simulink model "HDLModulatorFull"  (R2024a)
settings: Solver=FixedStepDiscrete  StartTime=0.0  StopTime=stopTime  RelTol=1e-3
values from neighbouring files (symbols this model uses):
  dataSymbols = [ ... (first row only)    [testModulatorFull.m]
undefined symbols (not defined in the file or in its folder): CONST
libraries: hdlsllib x10, dspsrcs4 x9, simulink x2, HDL_ieee_8021513 x2, whdlutilities x1
settings Model: DataTypeOverride=Off  SimulationMode=accelerator  Creator=cotti  LastModifiedBy=cotti
settings OptimizationCC: BlockReduction=off  ConditionallyExecuteInputs=off  DefaultParameterBehavior=Inlined  InheritOutputTypeSmallerThanSingle=on
settings DebuggingCC: AlgebraicLoopMsg=error  ArtificialAlgebraicLoopMsg=error  SingleTaskRateTransMsg=error  UnconnectedInputMsg=warning  UnconnectedOutputMsg=warning  UnconnectedLineMsg=warning
settings HardwareCC: ProdBitPerPointer=32  ProdBitPerSizeT=32  ProdBitPerPtrDiffT=32  ProdLargestAtomicFloat=None  ProdIntDivRoundTo=Undefined  ProdEndianess=Unspecified  ProdWordSize=32  ProdHWDeviceType=ASIC/FPGA->ASIC/FPGA  TargetBitPerLong=64  TargetBitPerPointer=64  TargetBitPerSizeT=64  TargetBitPerPtrDiffT=64  TargetLongLongMode=on  TargetIntDivRoundTo=Zero  TargetEndianess=LittleEndian  TargetWordSize=64  TargetHWDeviceType=Custom Processor->MATLAB Host Computer  ProdEqTarget=off

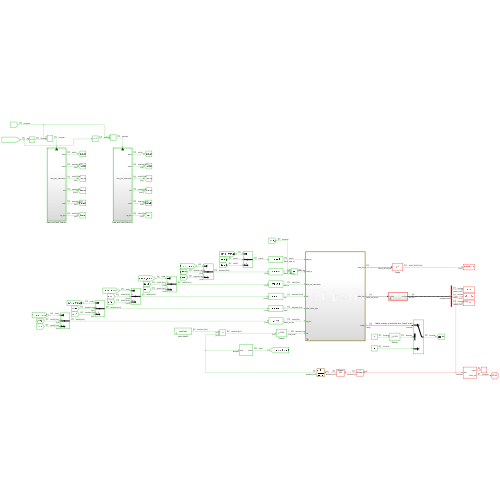
[thumbnail: Simulink's stored preview of the top-level diagram]
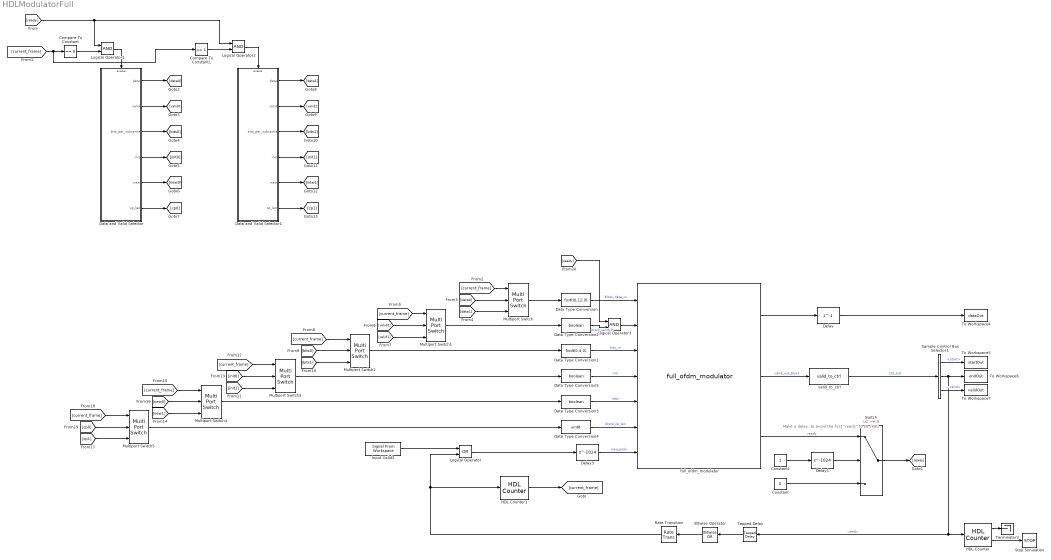
== system HDLModulatorFull ==
  note: Make a delay, to avoid the first "ready" to be read
  Bitwise Operator : simulink/Logic and Bit Operations/Bitwise Operator  logicop=OR  UseBitMask=off  BitMask=bin2dec('11011001')  BitMaskRealWorld=Stored Integer
      settings: LibrarySourceBlock=|
      | hdlsllib/Logic and Bit
      | Operations/Bitwise
      | Operator
  Compare To Constant : hdlsllib/Logic and Bit Operations/Compare To Constant  relop===  const=0  OutDataTypeStr=boolean
  Compare To Constant1 : hdlsllib/Logic and Bit Operations/Compare To Constant  relop===  const=1  OutDataTypeStr=boolean
  Constant : Constant  Value=0  OutDataTypeStr=boolean  SampleTime=1/CONST.fPHY
  Constant1 : Constant  OutDataTypeStr=boolean  SampleTime=1/CONST.fPHY
  Data Type Conversion : DataTypeConversion  OutDataTypeStr=fixdt(0,12,0)  SaturateOnIntegerOverflow=off  RndMeth=Floor  LockScale=on
  Data Type Conversion1 : DataTypeConversion  OutDataTypeStr=fixdt(0,4,0)  SaturateOnIntegerOverflow=off  RndMeth=Floor  LockScale=on
  Data Type Conversion2 : DataTypeConversion  OutDataTypeStr=boolean  SaturateOnIntegerOverflow=off  RndMeth=Floor  LockScale=on
  Data Type Conversion3 : DataTypeConversion  OutDataTypeStr=boolean  SaturateOnIntegerOverflow=off  RndMeth=Floor  LockScale=on
  Data Type Conversion4 : DataTypeConversion  OutDataTypeStr=uint8  SaturateOnIntegerOverflow=off  RndMeth=Floor  LockScale=on
  Data Type Conversion5 : DataTypeConversion  OutDataTypeStr=boolean  SaturateOnIntegerOverflow=off  RndMeth=Floor  LockScale=on
  Data and Valid Selector : Subsystem  TreatAsAtomicUnit=on
  Data and Valid Selector1 : Subsystem  TreatAsAtomicUnit=on
  Delay : Delay  DelayLength=1  InitialCondition=0  UseCircularBuffer=on
  Delay1 : Delay  DelayLength=1024  InitialCondition=0  UseCircularBuffer=on
  Delay3 : Delay  DelayLength=1024  InitialCondition=0  UseCircularBuffer=on
  HDL Counter : hdlsllib/Sources/HDL Counter  CountType=Count limited  CountInit=0  CountStep=1  CountMax=numberOfRepetitions  CountFromType=Initial value  CountFrom=0  CountResetPort=off  CountLoadPort=off  CountEnbPort=on  CountDirPort=off  CountHitOutputPort=on  CountDataType=Unsigned  CountWordLen=8  CountFracLen=0  CountSampTime=1
  HDL Counter1 : hdlsllib/Sources/HDL Counter  CountType=Free running  CountInit=0  CountStep=1  CountMax=25  CountFromType=Initial value  CountFrom=0  CountResetPort=off  CountLoadPort=off  CountEnbPort=on  CountDirPort=off  CountHitOutputPort=off  CountDataType=Unsigned  CountWordLen=8  CountFracLen=0  CountSampTime=1
  Input Valid3 : dspsrcs4/Signal From Workspace  X=newPsdu  Ts=1/CONST.fPHY  nsamps=1  OutputAfterFinalValue=Setting to zero  ignoreOrWarnInputAndFrameLengths=off  OutputFrames=off
  Logical Operator : Logic  Operator=OR  AllPortsSameDT=off  OutDataTypeStr=boolean
  Logical Operator1 : Logic  AllPortsSameDT=off  OutDataTypeStr=boolean
  Logical Operator2 : Logic  AllPortsSameDT=off  OutDataTypeStr=boolean
  Logical Operator3 : Logic  AllPortsSameDT=off  OutDataTypeStr=boolean
  Multiport Switch{,1..5} (6 alike) : MultiPortSwitch  DataPortOrder=Zero-based contiguous  Inputs=2  zeroidx=on  SaturateOnIntegerOverflow=off  InputSameDT=off
  Rate Transition : RateTransition  OutPortSampleTimeOpt=Multiple of input port sample time  OutPortSampleTimeMultiple=2
  Sample Control Bus Selector1 : whdlutilities/Sample Control Bus Selector  OutputSignals=start,end,valid
  Stop Simulation : Stop
  Switch : Switch  Criteria=u2 ~= 0  SaturateOnIntegerOverflow=off  InputSameDT=off
  Tapped Delay : simulink/Discrete/Tapped Delay  vinit=0.0  samptime=-1  NumDelays=2  DelayOrder=Oldest  includeCurrent=off
      settings: LibrarySourceBlock=hdlsllib/Discrete/Tapped Delay
  Terminator2 : Terminator
  To Workspace4 : ToWorkspace  VariableName=dataOut  SampleTime=1/CONST.fDAC
      settings: Save2DSignal=2-D array (concatenate along first dimension)
  To Workspace5 : ToWorkspace  VariableName=startOut  SampleTime=1/CONST.fDAC
      settings: Save2DSignal=2-D array (concatenate along first dimension)
  To Workspace6 : ToWorkspace  VariableName=endOut  SampleTime=1/CONST.fDAC
      settings: Save2DSignal=2-D array (concatenate along first dimension)
  To Workspace7 : ToWorkspace  VariableName=validOut  SampleTime=1/CONST.fDAC
      settings: Save2DSignal=2-D array (concatenate along first dimension)
  full_ofdm_modulator : HDL_ieee_8021513/full_ofdm_modulator  SystemSampleTime=-1  VariantActivationTime=update diagram  AllowFlexibleInterface=on  Latency=0  AutoFrameSizeCalculation=off
      settings: SourceProductName=HDL IEEE 8021513
  valid_to_ctrl : HDL_ieee_8021513/valid_to_ctrl  SystemSampleTime=-1  VariantActivationTime=update diagram  AllowFlexibleInterface=on  Latency=0  AutoFrameSizeCalculation=off
      settings: SourceProductName=HDL IEEE 8021513
  wires:
  full_ofdm_modulator/2 -> valid_to_ctrl/1  "valid_out_block"
  full_ofdm_modulator/1 -> Delay/1
  Sample Control Bus Selector1/3 -> To Workspace7/1  "<valid>"
  valid_to_ctrl/1 -> Sample Control Bus Selector1/1  "ctrl_out"
  Sample Control Bus Selector1/1 -> To Workspace5/1  "<start>"
  Sample Control Bus Selector1/2 -> Tapped Delay/1, HDL Counter/1, To Workspace6/1  "<end>"
  Data Type Conversion1/1 -> full_ofdm_modulator/3  "bits_in"
  Data Type Conversion4/1 -> full_ofdm_modulator/6  "block_cp_len"
  Data Type Conversion/1 -> full_ofdm_modulator/1  "block_data_in"
  Data Type Conversion3/1 -> full_ofdm_modulator/5  "new"
  Data Type Conversion5/1 -> full_ofdm_modulator/4  "init"
  Delay/1 -> To Workspace4/1
  HDL Counter/1 -> Terminator2/1
  HDL Counter/2 -> Stop Simulation/1
  full_ofdm_modulator/3 -> Switch/1  "ready"
  Constant/1 -> Switch/3
  Constant1/1 -> Delay1/1
  Delay1/1 -> Switch/2
  Rate Transition/1 -> Logical Operator/2, HDL Counter1/1
  Tapped Delay/1 -> Bitwise Operator/1
  Bitwise Operator/1 -> Rate Transition/1
  Input Valid3/1 -> Logical Operator/1
  Delay3/1 -> full_ofdm_modulator/7  "new_psdu"
  Logical Operator/1 -> Delay3/1
  HDL Counter1/1 -> [current_frame]
  Switch/1 -> [ready]
  Data and Valid Selector/1(data) -> [data0]
  Data and Valid Selector/2(valid) -> [valid0]
  Data and Valid Selector/3(bits_per_subcarrier) -> [bits0]
  Data and Valid Selector/4(init) -> [init0]
  Data and Valid Selector/5(new) -> [new0]
  Data and Valid Selector/6(cp_len) -> [cp0]
  Data and Valid Selector1/1(data) -> [data1]
  Data and Valid Selector1/2(valid) -> [valid1]
  Data and Valid Selector1/3(bits_per_subcarrier) -> [bits1]
  Data and Valid Selector1/4(init) -> [init1]
  Data and Valid Selector1/5(new) -> [new1]
  Data and Valid Selector1/6(cp_len) -> [cp1]
  [current_frame] -> Compare To Constant1/1, Compare To Constant/1
  Compare To Constant/1 -> Logical Operator1/2
  [ready] -> Logical Operator2/1, Logical Operator1/1
  Compare To Constant1/1 -> Logical Operator2/2
  Logical Operator2/1 -> Data and Valid Selector1/Enable
  Logical Operator1/1 -> Data and Valid Selector/Enable
  [current_frame] -> Multiport Switch/1
  [data0] -> Multiport Switch/2
  [data1] -> Multiport Switch/3
  Multiport Switch/1 -> Data Type Conversion/1
  [valid1] -> Multiport Switch1/3
  [valid0] -> Multiport Switch1/2
  Multiport Switch1/1 -> Data Type Conversion2/1
  [current_frame] -> Multiport Switch1/1
  [bits1] -> Multiport Switch2/3
  [bits0] -> Multiport Switch2/2
  Multiport Switch2/1 -> Data Type Conversion1/1
  [current_frame] -> Multiport Switch2/1
  [init0] -> Multiport Switch3/2
  [current_frame] -> Multiport Switch3/1
  [init1] -> Multiport Switch3/3
  Multiport Switch3/1 -> Data Type Conversion5/1
  [new0] -> Multiport Switch4/2
  [current_frame] -> Multiport Switch4/1
  [new1] -> Multiport Switch4/3
  Multiport Switch4/1 -> Data Type Conversion3/1
  [cp0] -> Multiport Switch5/2
  [current_frame] -> Multiport Switch5/1
  [cp1] -> Multiport Switch5/3
  Multiport Switch5/1 -> Data Type Conversion4/1
  Logical Operator3/1 -> full_ofdm_modulator/2
  Data Type Conversion2/1 -> Logical Operator3/2  "block_valid_in"
  [ready] -> Logical Operator3/1

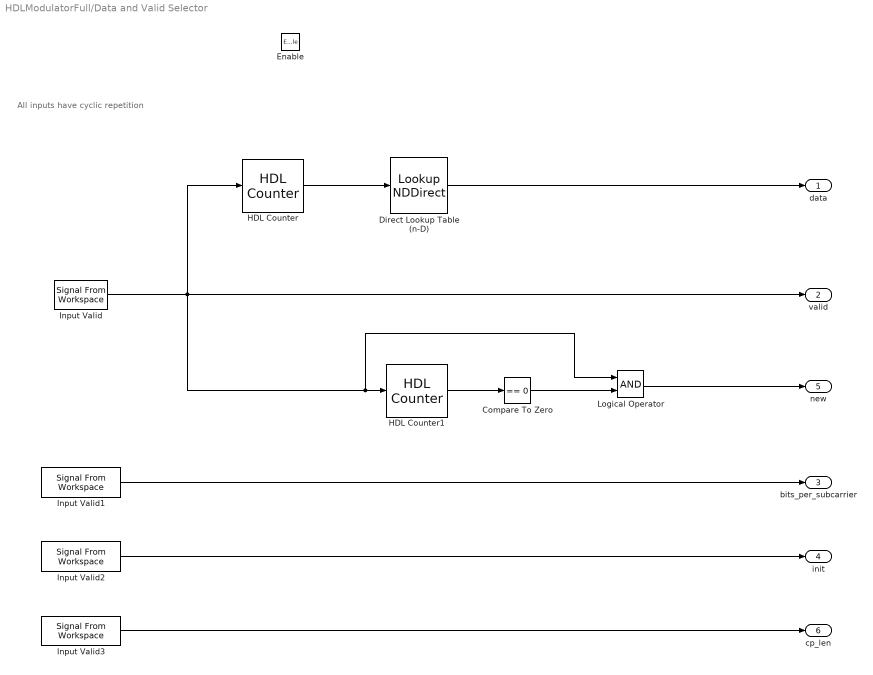
== system HDLModulatorFull/Data and Valid Selector ==
  note: All inputs have cyclic repetition
  Enable : EnablePort
  Compare To Zero : hdlsllib/Logic and Bit Operations/Compare To Zero  relop===  OutDataTypeStr=boolean
  Direct Lookup Table (n-D) : LookupNDDirect  NumberOfTableDimensions=1  Table=dataSymbols  DiagnosticForOutOfRangeInput=Error  TableDataTypeStr=fixdt(0,12,0)
  HDL Counter : hdlsllib/Sources/HDL Counter  CountType=Count limited  CountInit=0  CountStep=1  CountMax=length(dataSymbols) -1  CountFromType=Initial value  CountFrom=0  CountResetPort=off  CountLoadPort=off  CountEnbPort=on  CountDirPort=off  CountHitOutputPort=off  CountDataType=Unsigned  CountWordLen=nextpow2(length(dataSymbols))  CountFracLen=0  CountSampTime=1
  HDL Counter1 : hdlsllib/Sources/HDL Counter  CountType=Count limited  CountInit=0  CountStep=1  CountMax=CONST.numDataCarriers-1  CountFromType=Initial value  CountFrom=0  CountResetPort=off  CountLoadPort=off  CountEnbPort=on  CountDirPort=off  CountHitOutputPort=off  CountDataType=Unsigned  CountWordLen=nextpow2(CONST.numDataCarriers)  CountFracLen=0  CountSampTime=1
  Input Valid : dspsrcs4/Signal From Workspace  X=validIn  Ts=1/CONST.fPHY  nsamps=1  OutputAfterFinalValue=Setting to zero  ignoreOrWarnInputAndFrameLengths=off  OutputFrames=off
  Input Valid1 : dspsrcs4/Signal From Workspace  X=bitsPerSubcarrier  Ts=1/CONST.fPHY  nsamps=1  OutputAfterFinalValue=Setting to zero  ignoreOrWarnInputAndFrameLengths=off  OutputFrames=off
  Input Valid2 : dspsrcs4/Signal From Workspace  X=init  Ts=1/CONST.fPHY  nsamps=1  OutputAfterFinalValue=Setting to zero  ignoreOrWarnInputAndFrameLengths=off  OutputFrames=off
  Input Valid3 : dspsrcs4/Signal From Workspace  X=cpLen  Ts=1/CONST.fPHY  nsamps=1  OutputAfterFinalValue=Setting to zero  ignoreOrWarnInputAndFrameLengths=off  OutputFrames=off
  Logical Operator : Logic  AllPortsSameDT=off  OutDataTypeStr=boolean
  data : Outport  InitialOutput=0  VectorParamsAs1DForOutWhenUnconnected=off
  valid : Outport  Port=2  InitialOutput=0  VectorParamsAs1DForOutWhenUnconnected=off
  bits_per_subcarrier : Outport  Port=3  VectorParamsAs1DForOutWhenUnconnected=off
  init : Outport  Port=4  VectorParamsAs1DForOutWhenUnconnected=off
  new : Outport  Port=5  VectorParamsAs1DForOutWhenUnconnected=off
  cp_len : Outport  Port=6  VectorParamsAs1DForOutWhenUnconnected=off
  wires:
  HDL Counter/1 -> Direct Lookup Table (n-D)/1
  HDL Counter1/1 -> Compare To Zero/1
  Compare To Zero/1 -> Logical Operator/2
  Direct Lookup Table (n-D)/1 -> data/1
  Input Valid/1 -> valid/1, HDL Counter/1, Logical Operator/1, HDL Counter1/1
  Logical Operator/1 -> new/1
  Input Valid1/1 -> bits_per_subcarrier/1
  Input Valid2/1 -> init/1
  Input Valid3/1 -> cp_len/1

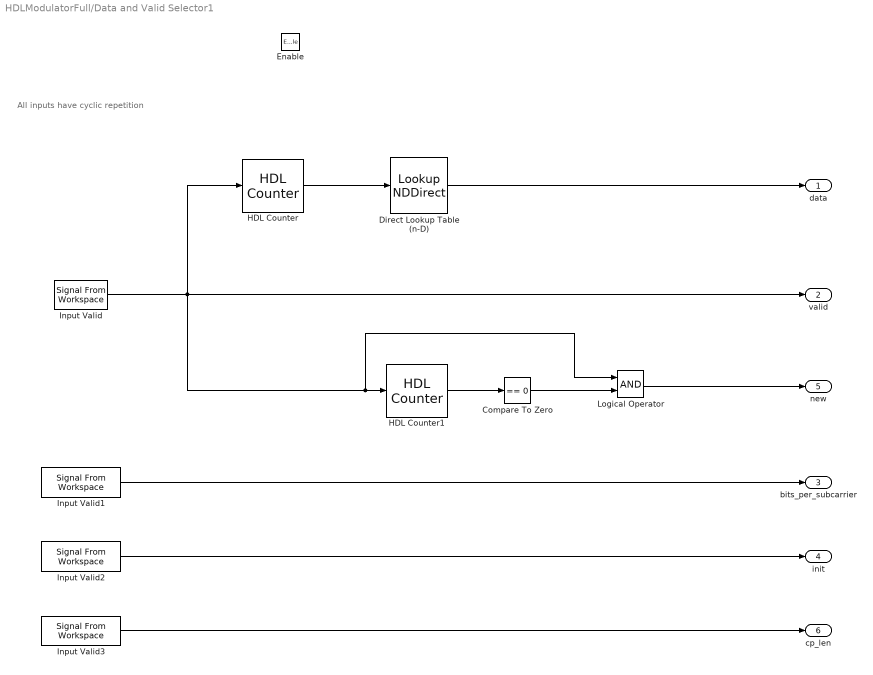
== system HDLModulatorFull/Data and Valid Selector1 ==
  note: All inputs have cyclic repetition
  Enable : EnablePort
  Compare To Zero : hdlsllib/Logic and Bit Operations/Compare To Zero  relop===  OutDataTypeStr=boolean
  Direct Lookup Table (n-D) : LookupNDDirect  NumberOfTableDimensions=1  Table=dataSymbols  DiagnosticForOutOfRangeInput=Error  TableDataTypeStr=fixdt(0,12,0)
  HDL Counter : hdlsllib/Sources/HDL Counter  CountType=Count limited  CountInit=0  CountStep=1  CountMax=length(dataSymbols) -1  CountFromType=Initial value  CountFrom=0  CountResetPort=off  CountLoadPort=off  CountEnbPort=on  CountDirPort=off  CountHitOutputPort=off  CountDataType=Unsigned  CountWordLen=nextpow2(length(dataSymbols))  CountFracLen=0  CountSampTime=1
  HDL Counter1 : hdlsllib/Sources/HDL Counter  CountType=Count limited  CountInit=0  CountStep=1  CountMax=CONST.numDataCarriers-1  CountFromType=Initial value  CountFrom=0  CountResetPort=off  CountLoadPort=off  CountEnbPort=on  CountDirPort=off  CountHitOutputPort=off  CountDataType=Unsigned  CountWordLen=nextpow2(CONST.numDataCarriers)  CountFracLen=0  CountSampTime=1
  Input Valid : dspsrcs4/Signal From Workspace  X=validIn  Ts=1/CONST.fPHY  nsamps=1  OutputAfterFinalValue=Setting to zero  ignoreOrWarnInputAndFrameLengths=off  OutputFrames=off
  Input Valid1 : dspsrcs4/Signal From Workspace  X=bitsPerSubcarrier  Ts=1/CONST.fPHY  nsamps=1  OutputAfterFinalValue=Setting to zero  ignoreOrWarnInputAndFrameLengths=off  OutputFrames=off
  Input Valid2 : dspsrcs4/Signal From Workspace  X=init  Ts=1/CONST.fPHY  nsamps=1  OutputAfterFinalValue=Setting to zero  ignoreOrWarnInputAndFrameLengths=off  OutputFrames=off
  Input Valid3 : dspsrcs4/Signal From Workspace  X=cpLen  Ts=1/CONST.fPHY  nsamps=1  OutputAfterFinalValue=Setting to zero  ignoreOrWarnInputAndFrameLengths=off  OutputFrames=off
  Logical Operator : Logic  AllPortsSameDT=off  OutDataTypeStr=boolean
  data : Outport  InitialOutput=0  VectorParamsAs1DForOutWhenUnconnected=off
  valid : Outport  Port=2  InitialOutput=0  VectorParamsAs1DForOutWhenUnconnected=off
  bits_per_subcarrier : Outport  Port=3  VectorParamsAs1DForOutWhenUnconnected=off
  init : Outport  Port=4  VectorParamsAs1DForOutWhenUnconnected=off
  new : Outport  Port=5  VectorParamsAs1DForOutWhenUnconnected=off
  cp_len : Outport  Port=6  VectorParamsAs1DForOutWhenUnconnected=off
  wires:
  HDL Counter/1 -> Direct Lookup Table (n-D)/1
  HDL Counter1/1 -> Compare To Zero/1
  Compare To Zero/1 -> Logical Operator/2
  Direct Lookup Table (n-D)/1 -> data/1
  Input Valid/1 -> valid/1, HDL Counter/1, Logical Operator/1, HDL Counter1/1
  Logical Operator/1 -> new/1
  Input Valid1/1 -> bits_per_subcarrier/1
  Input Valid2/1 -> init/1
  Input Valid3/1 -> cp_len/1
